simulink model "SRManL4_ZADANIE1_MODEL"  (R2018a)
settings: Solver=ode45  StartTime=0.0  StopTime=tend  MaxStep=Tp  RelTol=1e-3
values from neighbouring files (symbols this model uses):
  D = diag([d1 d2])    [SRManL4_ZADANIE1_SKRYPT.m]
  eta = diag([eta1; eta2])    [SRManL4_ZADANIE1_SKRYPT.m]
  initConditionsPos = [0; 0]    [SRManL4_ZADANIE1_SKRYPT.m]
  initConditionsVel = [0; 0]    [SRManL4_ZADANIE1_SKRYPT.m]
  invR = inv(R)    [SRManL4_ZADANIE1_SKRYPT.m]
  Km = diag([km1; km2])    [SRManL4_ZADANIE1_SKRYPT.m]
  Lambda = diag([lambda1 lambda2])    [SRManL4_ZADANIE1_SKRYPT.m]
  omega1 = 0.6    [SRManL4_ZADANIE1_SKRYPT.m]
  omega2 = 0.7    [SRManL4_ZADANIE1_SKRYPT.m]
  Qd01 = 0.0025    [SRManL4_ZADANIE1_SKRYPT.m]
  Qd02 = 0.0025    [SRManL4_ZADANIE1_SKRYPT.m]
  Qd1 = 1    [SRManL4_ZADANIE1_SKRYPT.m]
  Qd11 = 0.0020    (= 0.002)    [SRManL4_ZADANIE1_SKRYPT.m]
  Qd12 = 0.002    [SRManL4_ZADANIE1_SKRYPT.m]
  Qd1const = 1    [SRManL4_ZADANIE1_SKRYPT.m]
  Qd2 = 1    [SRManL4_ZADANIE1_SKRYPT.m]
  Qd21 = 0.0015    [SRManL4_ZADANIE1_SKRYPT.m]
  Qd22 = 0.0015    [SRManL4_ZADANIE1_SKRYPT.m]
  Qd2const = 1    [SRManL4_ZADANIE1_SKRYPT.m]
  Qd31 = 0.001    [SRManL4_ZADANIE1_SKRYPT.m]
  Qd32 = 0.001    [SRManL4_ZADANIE1_SKRYPT.m]
  u1max = 24    [SRManL4_ZADANIE1_SKRYPT.m]
libraries: dsppolyfun x6, simulink x2
settings Model: Creator=szymon  LastModifiedBy=szymon

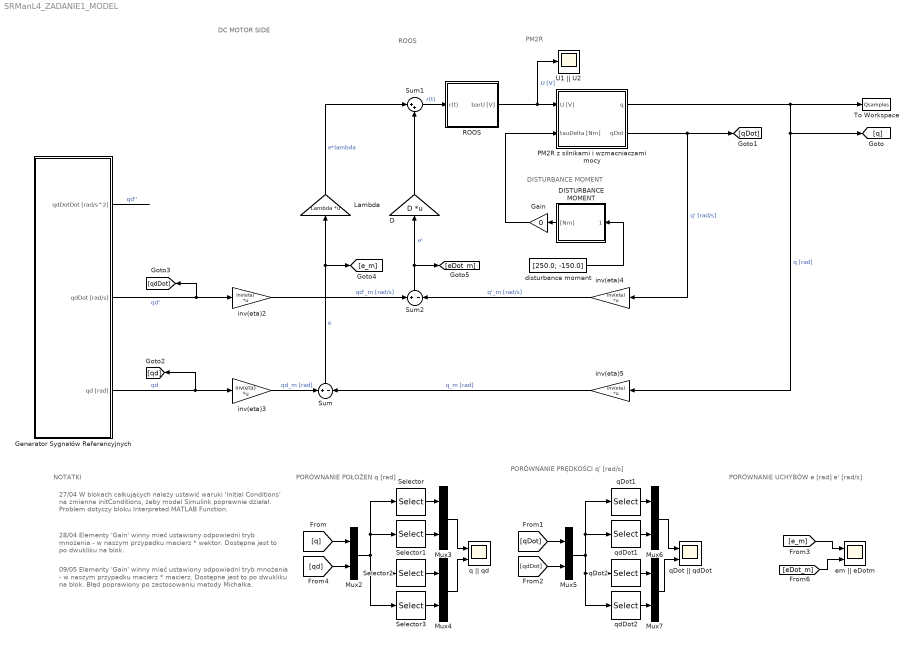
== system SRManL4_ZADANIE1_MODEL ==
  note: DC MOTOR SIDE
  note: PORÓWNANIE POŁOŻEŃ
      | q [rad]
  note: NOTATKI
  note: 27/04 W blokach całkujących należy ustawić waruki
      | 'Initial Conditions' na zmienne initConditions, żeby model
      | Simulink poprawnie działał. Problem dotyczy bloku
      | Interpreted MATLAB Function.
  note: 28/04 Elementy 'Gain' winny mieć ustawiony odpowiedni tryb
      | mnożenia - w naszym przypadku macierz * wektor.
      | Dostępne jest to po dwukliku na blok.
  note: PORÓWNANIE PRĘDKOŚCI
      | q' [rad/s]
  note: 09/05 Elementy 'Gain' winny mieć ustawiony odpowiedni tryb
      | mnożenia - w naszym przypadku macierz * macierz.
      | Dostępne jest to po dwukliku na blok. Błąd poprawiony po
      | zastosowaniu metody Michałka.
  note: PORÓWNANIE UCHYBÓW
      | e  [rad]
      | e' [rad/s]
  note: ROOS
  note: PM2R
  note: DISTURBANCE MOMENT
  D : Gain  Gain=D  Multiplication=Matrix(K*u) (u vector)
  DISTURBANCE MOMENT : Subsystem
  Gain : Gain  Gain=0
  Generator Sygnałów Referencyjnych : Subsystem
  Lambda : Gain  Gain=Lambda  Multiplication=Matrix(K*u) (u vector)
  Mux{2..7} (6 alike) : Mux  Inputs=2
  PM2R z silnikami i wzmacniaczami mocy : Subsystem
  ROOS : Subsystem
  Selector : Selector  InputPortWidth=4  IndexOptions=Index vector (dialog)  Indices=[1]  OutputSizes=1
  Selector1 : Selector  InputPortWidth=4  IndexOptions=Index vector (dialog)  Indices=[3]  OutputSizes=1
  Selector2 : Selector  InputPortWidth=4  IndexOptions=Index vector (dialog)  Indices=[2]  OutputSizes=1
  Selector3 : Selector  InputPortWidth=4  IndexOptions=Index vector (dialog)  Indices=[4]  OutputSizes=1
  Sum : Sum  Inputs=+-
  Sum1 : Sum  Inputs=|++
  Sum2 : Sum  Inputs=+-
  To Workspace : ToWorkspace  VariableName=Qsamples  SampleTime=-1
  U1 || U2 : Scope
  disturbance moment : Constant  Value=[250.0; -150.0]
  em || eDotm : Scope  NumInputPorts=2
  inv(eta){2..5} (4 alike) : Gain  Gain=inv(eta)  Multiplication=Matrix(K*u)
  q || qd : Scope  NumInputPorts=2
  qDot || qdDot : Scope  NumInputPorts=2
  qDot1 : Selector  InputPortWidth=4  IndexOptions=Index vector (dialog)  Indices=[1]  OutputSizes=1
  qDot2 : Selector  InputPortWidth=4  IndexOptions=Index vector (dialog)  Indices=[2]  OutputSizes=1
  qdDot1 : Selector  InputPortWidth=4  IndexOptions=Index vector (dialog)  Indices=[3]  OutputSizes=1
  qdDot2 : Selector  InputPortWidth=4  IndexOptions=Index vector (dialog)  Indices=[4]  OutputSizes=1
  wires:
  PM2R z silnikami i wzmacniaczami mocy/2(qDot) -> inv(eta)4/1, [qDot]  "q' [rad/s]"
  PM2R z silnikami i wzmacniaczami mocy/1(q) -> inv(eta)5/1, [q], To Workspace/1  "q [rad]"
  [q] -> Mux2/1
  [qd] -> Mux2/2
  Selector/1 -> Mux3/1
  Selector1/1 -> Mux3/2
  Selector2/1 -> Mux4/1
  Selector3/1 -> Mux4/2
  Mux2/1 -> Selector3/1, Selector2/1, Selector1/1, Selector/1
  Mux3/1 -> q || qd/1
  Mux4/1 -> q || qd/2
  qDot2/1 -> Mux7/1
  Mux6/1 -> qDot || qdDot/1
  Mux7/1 -> qDot || qdDot/2
  qdDot2/1 -> Mux7/2
  [qDot] -> Mux5/1
  qdDot1/1 -> Mux6/2
  [qdDot] -> Mux5/2
  qDot1/1 -> Mux6/1
  Mux5/1 -> qdDot2/1, qDot2/1, qdDot1/1, qDot1/1
  Generator Sygnałów Referencyjnych/2(qdDot [rad/s]) -> [qdDot], inv(eta)2/1  "qd'"
  Generator Sygnałów Referencyjnych/1(qdDotDot [rad/s^2]) -> ?  "qd''"
  inv(eta)2/1 -> Sum2/1  "qd'_m [rad/s]"
  ROOS/1(barU [V]) -> U1 || U2/1, PM2R z silnikami i wzmacniaczami mocy/1(U [V])  "U [V]"
  [e_m] -> em || eDotm/1
  inv(eta)4/1 -> Sum2/2  "q'_m [rad/s]"
  inv(eta)5/1 -> Sum/2  "q_m [rad]"
  inv(eta)3/1 -> Sum/1  "qd_m [rad]"
  Generator Sygnałów Referencyjnych/3(qd [rad]) -> [qd], inv(eta)3/1  "qd"
  [eDot_m] -> em || eDotm/2
  Sum1/1 -> ROOS/1(r(t))  "r(t)"
  Sum2/1 -> D/1, [eDot_m]  "e'"
  Lambda/1 -> Sum1/1  "e*lambda"
  D/1 -> Sum1/2
  Sum/1 -> [e_m], Lambda/1  "e"
  DISTURBANCE MOMENT/1("[Nm]") -> Gain/1
  disturbance moment/1 -> DISTURBANCE MOMENT/1(in [Nm])
  Gain/1 -> PM2R z silnikami i wzmacniaczami mocy/2(tauDelta [Nm])

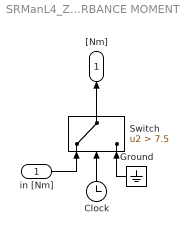
== system SRManL4_ZADANIE1_MODEL/DISTURBANCE MOMENT ==
  in [Nm] : Inport
  Clock : Clock
  Ground : Ground
  Switch : Switch  Criteria=u2 > Threshold  Threshold=7.5
  "[Nm]" : Outport
  wires:
  Clock/1 -> Switch/2
  Ground/1 -> Switch/3
  in [Nm]/1 -> Switch/1
  Switch/1 -> "[Nm]"/1

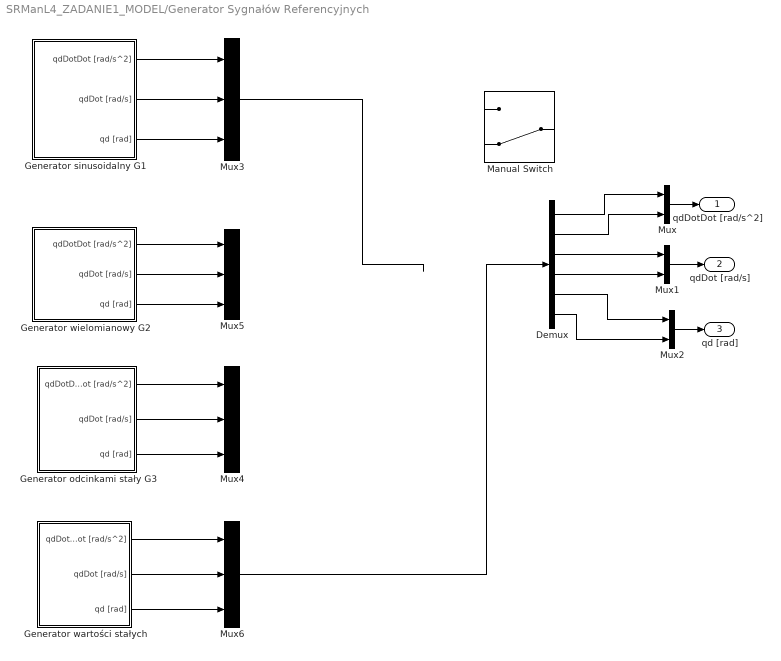
== system SRManL4_ZADANIE1_MODEL/Generator Sygnałów Referencyjnych ==
  Demux : Demux  Outputs=6
  "Generator odcinkami stały G3 " : Subsystem
  Generator sinusoidalny G1 : Subsystem
  Generator wielomianowy G2 : Subsystem
  Generator wartości stałych : Subsystem
  Manual Switch : ManualSwitch  CurrentSetting=0
  Mux : Mux  Inputs=2
  Mux1 : Mux  Inputs=2
  Mux2 : Mux  Inputs=2
  Mux{3..6} (4 alike) : Mux  Inputs=3
  qdDotDot [rad/s^2] : Outport
  qdDot [rad/s] : Outport  Port=2
  qd [rad] : Outport  Port=3
  wires:
  Mux/1 -> qdDotDot [rad/s^2]/1
  Mux2/1 -> qd [rad]/1
  Mux1/1 -> qdDot [rad/s]/1
  Demux/1 -> Mux/1
  Demux/2 -> Mux/2
  Demux/3 -> Mux1/1
  Demux/4 -> Mux1/2
  Demux/5 -> Mux2/1
  Demux/6 -> Mux2/2
  Generator sinusoidalny G1/2(qdDot [rad/s]) -> Mux3/2
  Generator sinusoidalny G1/1(qdDotDot [rad/s^2]) -> Mux3/1
  Generator sinusoidalny G1/3(qd [rad]) -> Mux3/3
  "Generator odcinkami stały G3 "/1(qdDotDot [rad/s^2]) -> Mux4/1
  "Generator odcinkami stały G3 "/2(qdDot [rad/s]) -> Mux4/2
  "Generator odcinkami stały G3 "/3(qd [rad]) -> Mux4/3
  Generator wielomianowy G2/1(qdDotDot [rad/s^2]) -> Mux5/1
  Generator wielomianowy G2/2(qdDot [rad/s]) -> Mux5/2
  Generator wielomianowy G2/3(qd [rad]) -> Mux5/3
  Generator wartości stałych/1(qdDotDot [rad/s^2]) -> Mux6/1
  Generator wartości stałych/3(qd [rad]) -> Mux6/3
  Generator wartości stałych/2(qdDot [rad/s]) -> Mux6/2
  Mux3/1 -> ?
  Mux6/1 -> Demux/1

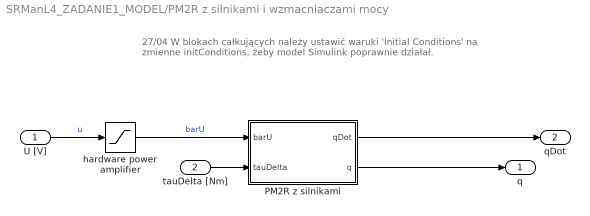
== system SRManL4_ZADANIE1_MODEL/PM2R z silnikami i wzmacniaczami mocy ==
  note: 27/04 W blokach całkujących należy ustawić waruki 'Initial Conditions' na
      | zmienne initConditions, żeby model Simulink poprawnie działał.
  U [V] : Inport
  tauDelta [Nm] : Inport  Port=2
  PM2R z silnikami : Subsystem
  hardware power amplifier : Saturate  UpperLimit=24.0  LowerLimit=-24.0
  q : Outport
  qDot : Outport  Port=2
  wires:
  U [V]/1 -> hardware power amplifier/1  "u"
  PM2R z silnikami/1(qDot) -> qDot/1
  PM2R z silnikami/2(q) -> q/1
  tauDelta [Nm]/1 -> PM2R z silnikami/2(tauDelta)
  hardware power amplifier/1 -> PM2R z silnikami/1(barU)  "barU"

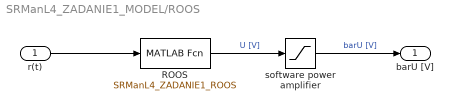
== system SRManL4_ZADANIE1_MODEL/ROOS ==
  r(t) : Inport
  ROOS : MATLABFcn  MATLABFcn=SRManL4_ZADANIE1_ROOS
  software power amplifier : Saturate  UpperLimit=u1max  LowerLimit=-u1max
  barU [V] : Outport
  wires:
  ROOS/1 -> software power amplifier/1  "U [V]"
  r(t)/1 -> ROOS/1
  software power amplifier/1 -> barU [V]/1  "barU [V]"

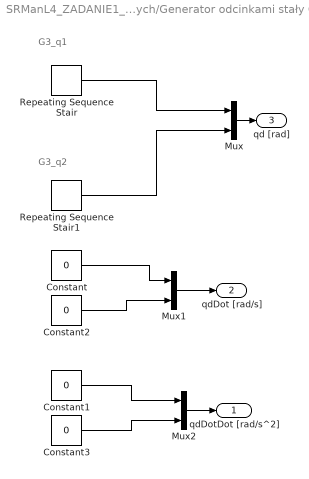
== system SRManL4_ZADANIE1_MODEL/Generator Sygnałów Referencyjnych/Generator odcinkami stały G3  ==
  note: G3_q2
  note: G3_q1
  Constant{,1..3} (4 alike) : Constant  Value=0
  Mux : Mux  Inputs=2
  Mux1 : Mux  Inputs=2
  Mux2 : Mux  Inputs=2
  Repeating Sequence Stair : simulink/Sources/Repeating Sequence Stair  OutValues=[Qd1const 0 0 0 0 0].'  tsamp=Ta  OutMin=[]  OutMax=[]  OutDataTypeStr=double  OutputDataTypeScalingMode=double  OutDataType=fixdt(0,8)  ConRadixGroup=Best Precision: Vector-wise  OutScaling=2^-12
  Repeating Sequence Stair1 : simulink/Sources/Repeating Sequence Stair  OutValues=[Qd2const 0 0 0 0 0].'  tsamp=Tb  OutMin=[]  OutMax=[]  OutDataTypeStr=double  OutputDataTypeScalingMode=double  OutDataType=fixdt(0,8)  ConRadixGroup=Best Precision: Vector-wise  OutScaling=2^-12
  qdDotDot [rad/s^2] : Outport
  qdDot [rad/s] : Outport  Port=2
  qd [rad] : Outport  Port=3
  wires:
  Constant/1 -> Mux1/1
  Repeating Sequence Stair1/1 -> Mux/2
  Repeating Sequence Stair/1 -> Mux/1
  Mux/1 -> qd [rad]/1
  Constant1/1 -> Mux2/1
  Constant2/1 -> Mux1/2
  Constant3/1 -> Mux2/2
  Mux2/1 -> qdDotDot [rad/s^2]/1
  Mux1/1 -> qdDot [rad/s]/1

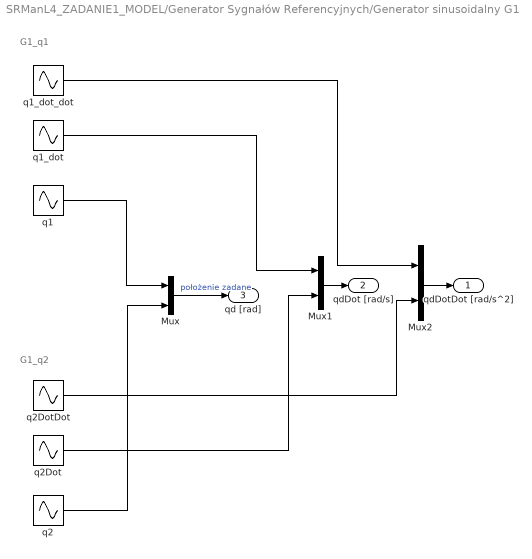
== system SRManL4_ZADANIE1_MODEL/Generator Sygnałów Referencyjnych/Generator sinusoidalny G1 ==
  note: G1_q1
  note: G1_q2
  Mux : Mux  Inputs=2
  Mux1 : Mux  Inputs=2
  Mux2 : Mux  Inputs=2
  "q1 " : Sin  Amplitude=Qd1  Frequency=omega1  SampleTime=0
  q1_dot : Sin  Amplitude=omega1*Qd1  Frequency=omega1  Phase=pi/2  SampleTime=0
  "q1_dot_dot " : Sin  Amplitude=-omega1^2*Qd1  Frequency=omega1  SampleTime=0
  q2 : Sin  Amplitude=Qd2  Frequency=omega2  SampleTime=0
  q2Dot : Sin  Amplitude=omega2*Qd2  Frequency=omega2  Phase=pi/2  SampleTime=0
  "q2DotDot " : Sin  Amplitude=-omega2^2*Qd2  Frequency=omega2  SampleTime=0
  qdDotDot [rad/s^2] : Outport
  qdDot [rad/s] : Outport  Port=2
  qd [rad] : Outport  Port=3
  wires:
  Mux1/1 -> qdDot [rad/s]/1
  Mux2/1 -> qdDotDot [rad/s^2]/1
  q2/1 -> Mux/2
  "q1 "/1 -> Mux/1
  Mux/1 -> qd [rad]/1  "położenie zadane"
  "q1_dot_dot "/1 -> Mux2/1
  q1_dot/1 -> Mux1/1
  "q2DotDot "/1 -> Mux2/2
  q2Dot/1 -> Mux1/2

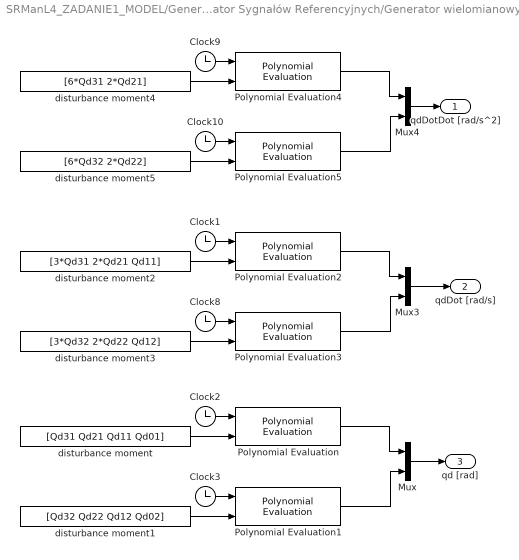
== system SRManL4_ZADANIE1_MODEL/Generator Sygnałów Referencyjnych/Generator wielomianowy G2 ==
  Clock{1..3,8..10} (6 alike) : Clock
  Mux : Mux  Inputs=2
  Mux3 : Mux  Inputs=2
  Mux4 : Mux  Inputs=2
  Polynomial Evaluation{,1..5} (6 alike) : dsppolyfun/Polynomial Evaluation  useConstCoeffs=off  constCoeffs=[5 4 3 2 1]
      settings: SourceProductName=DSP System Toolbox  SourceProductBaseCode=DS
  disturbance moment : Constant  Value=[Qd31 Qd21 Qd11 Qd01]
  disturbance moment1 : Constant  Value=[Qd32 Qd22 Qd12 Qd02]
  disturbance moment2 : Constant  Value=[3*Qd31 2*Qd21 Qd11]
  disturbance moment3 : Constant  Value=[3*Qd32 2*Qd22 Qd12]
  disturbance moment4 : Constant  Value=[6*Qd31 2*Qd21]
  disturbance moment5 : Constant  Value=[6*Qd32 2*Qd22]
  qdDotDot [rad/s^2] : Outport
  qdDot [rad/s] : Outport  Port=2
  qd [rad] : Outport  Port=3
  wires:
  Mux/1 -> qd [rad]/1
  disturbance moment/1 -> Polynomial Evaluation/2
  disturbance moment1/1 -> Polynomial Evaluation1/2
  Polynomial Evaluation/1 -> Mux/1
  Polynomial Evaluation1/1 -> Mux/2
  Clock2/1 -> Polynomial Evaluation/1
  Clock3/1 -> Polynomial Evaluation1/1
  Mux3/1 -> qdDot [rad/s]/1
  Clock1/1 -> Polynomial Evaluation2/1
  disturbance moment3/1 -> Polynomial Evaluation3/2
  Polynomial Evaluation2/1 -> Mux3/1
  disturbance moment2/1 -> Polynomial Evaluation2/2
  Polynomial Evaluation3/1 -> Mux3/2
  Clock8/1 -> Polynomial Evaluation3/1
  Clock10/1 -> Polynomial Evaluation5/1
  Polynomial Evaluation5/1 -> Mux4/2
  Polynomial Evaluation4/1 -> Mux4/1
  disturbance moment5/1 -> Polynomial Evaluation5/2
  Clock9/1 -> Polynomial Evaluation4/1
  disturbance moment4/1 -> Polynomial Evaluation4/2
  Mux4/1 -> qdDotDot [rad/s^2]/1

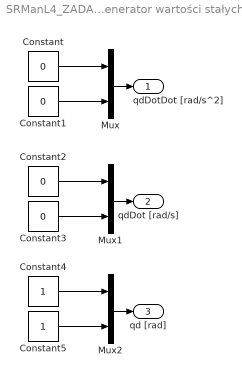
== system SRManL4_ZADANIE1_MODEL/Generator Sygnałów Referencyjnych/Generator wartości stałych ==
  Constant{,1..3} (4 alike) : Constant  Value=0
  Constant4 : Constant
  Constant5 : Constant
  Mux : Mux  Inputs=2
  Mux1 : Mux  Inputs=2
  Mux2 : Mux  Inputs=2
  qdDotDot [rad/s^2] : Outport
  qdDot [rad/s] : Outport  Port=2
  qd [rad] : Outport  Port=3
  wires:
  Constant/1 -> Mux/1
  Mux/1 -> qdDotDot [rad/s^2]/1
  Constant1/1 -> Mux/2
  Constant2/1 -> Mux1/1
  Constant3/1 -> Mux1/2
  Mux1/1 -> qdDot [rad/s]/1
  Constant4/1 -> Mux2/1
  Constant5/1 -> Mux2/2
  Mux2/1 -> qd [rad]/1

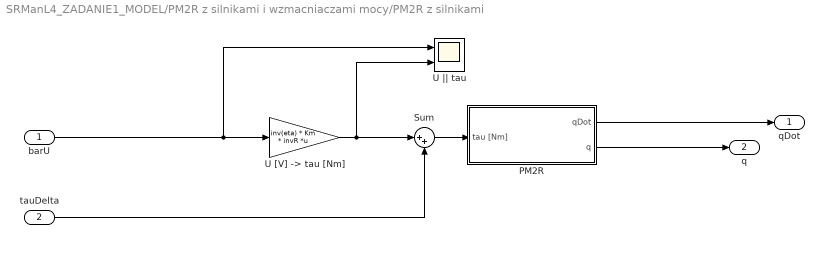
== system SRManL4_ZADANIE1_MODEL/PM2R z silnikami i wzmacniaczami mocy/PM2R z silnikami ==
  barU : Inport
  tauDelta : Inport  Port=2
  PM2R : Subsystem
  Sum : Sum  Inputs=|++
  "U [V] -> tau [Nm]" : Gain  Gain=inv(eta) * Km * invR  Multiplication=Matrix(K*u)
  U || tau : Scope  NumInputPorts=2
  qDot : Outport
  q : Outport  Port=2
  wires:
  PM2R/2(q) -> q/1
  PM2R/1(qDot) -> qDot/1
  barU/1 -> U || tau/1, "U [V] -> tau [Nm]"/1
  Sum/1 -> PM2R/1(tau [Nm])
  tauDelta/1 -> Sum/2
  "U [V] -> tau [Nm]"/1 -> U || tau/2, Sum/1

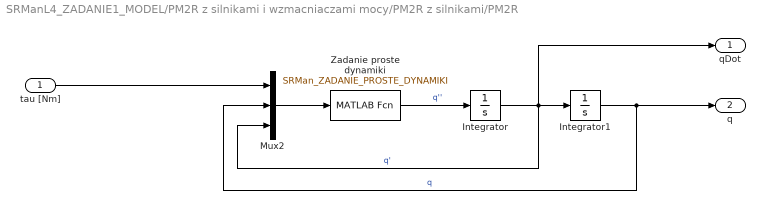
== system SRManL4_ZADANIE1_MODEL/PM2R z silnikami i wzmacniaczami mocy/PM2R z silnikami/PM2R ==
  tau [Nm] : Inport
  Integrator : Integrator  InitialCondition=initConditionsVel
  Integrator1 : Integrator  InitialCondition=initConditionsPos
  Mux2 : Mux  Inputs=3
  Zadanie proste dynamiki : MATLABFcn  MATLABFcn=SRMan_ZADANIE_PROSTE_DYNAMIKI
  qDot : Outport
  q : Outport  Port=2
  wires:
  Mux2/1 -> Zadanie proste dynamiki/1
  Integrator1/1 -> q/1, Mux2/2  "q"
  Integrator/1 -> Mux2/3, Integrator1/1, qDot/1  "q'"
  Zadanie proste dynamiki/1 -> Integrator/1  "q''"
  tau [Nm]/1 -> Mux2/1
